simulink model "LGS_allFaultsDeselected"  (R2019b)
settings: Solver=FixedStepDiscrete  StartTime=0.0  StopTime=45.0  FixedStep=0.1  RelTol=1e-3
model workspace (MAT data in the model file):
  fipData{1} = [0; 0]
  fipData{2} = [0; 0]
  fipData{3} = [0; 0]
  fipData{4} = [0; 0]
  fipData{5} = [0; 0]
  fipData{6} = [0; 0]
  fipData{7} = [0; 0]
  fipData{8} = [0; 0]
  fipData{9} = [0; 0]
  fipData{10} = [0; 0]
  fipData{11} = [0; 0]
  fipData{12} = [0; 0]
  fipData{13} = [0; 0]
  fipData{14} = [0; 0]
  fipData{15} = [0; 0]
  fipData{16} = [0; 0]
  fipData{17} = [0; 0]
  fipData{18} = [0; 0]
  fipData{19} = [0; 0]
  fipData{20} = [0; 0]
  fipData{21} = [0; 0]
  fipData{22} = [0; 0]
  fipData{23} = [0; 0]
  fipData{24} = [0; 0]
  fipData{25} = [0; 0]
  fipData{26} = [0; 0]
  fipData{27} = [0; 0]
  fipData{28} = [0; 0]
  fipData{29} = [0; 0]
  fipData{30} = [0; 0]
  fipData{31} = [0; 0]
  fipData{32} = [0; 0]
  fipData{33} = [0; 0]
  fipData{34} = [0; 0]
  fipData{35} = [0; 0]
  fipData{36} = [0; 0]
  fipData{37} = [0; 0]
  fipData{38} = [0; 0]
  fipData{39} = [0; 0]
  fipData{40} = [0; 0]
  fipData{41} = [0; 0]
  fipData{42} = [0; 0]
  fipData{43} = [0; 0]
  fipData{44} = [0; 0]
  fipData{45} = [0; 0]
  fipData{46} = [0; 0]
  fipData{47} = [0; 0]
  fipData{48} = [0; 0]
  fipData{49} = [0; 0]
  fipData{50} = [0; 0]
  fipData{51} = [0; 0]
  fipData{52} = [0; 0]
  fipData{53} = [0; 0]
  fipData{54} = [0; 0]
  fipData{55} = [0; 0]
  fipData{56} = [0; 0]
  fipData{57} = [0; 0]
  fipData{58} = [0; 0]
  fipData{59} = [0; 0]
  fipData{60} = [0; 0]
  fipData{61} = [0; 0]
  fipData{62} = [0; 0]
  fipData{63} = [0; 0]
  fipData{64} = [0; 0]
  fipData{65} = [0; 0]
  fipData{66} = [0; 0]
  fipData{67} = [0; 0]
  fipData{68} = [0; 0]
  fipData{69} = [0; 0]
  fipData{70} = [0; 0]
  fipData{71} = [0; 0]
  fipData{72} = [0; 0]
  fipData{73} = [0; 0]
  fipData{74} = [0; 0]
  fipData{75} = [0; 0]
  fipData{76} = [0; 0]
  fipData{77} = [0; 0]
  fipData{78} = [0; 0]
  fipData{79} = [0; 0]
  fipData{80} = [0; 0]
  fipData{81} = [0; 0]
  fipData{82} = [0; 0]
  fipData{83} = [0; 0]
  fipData{84} = [0; 0]
  fipData{85} = [0; 0]
  fipData{86} = [0; 0]
  fipData{87} = [0; 0]
  fipData{88} = [0; 0]
  fipData{89} = [0; 0]
  fipData{90} = [0; 0]
  fipData{91} = [0; 0]
  fipData{92} = [0; 0]
  fipData{93} = [0; 0]
  fipData{94} = [0; 0]
  fipData{95} = [0; 0]
  fipData{96} = [0; 0]
  fipData{97} = [0; 0]
  fipData{98} = [0; 0]
  fipData{99} = [0; 0]
  fipData{100} = [0; 0]
  fipData{101} = [0; 0]
  fipData{102} = [0; 0]
  fipData{103} = [0; 0]
  fipData{104} = [0; 0]
  fipData{105} = [0; 0]
  fipData{106} = [0; 0]
  fipData{107} = [0; 0]
  fipData{108} = [0; 0]
  fipData{109} = [0; 0]
  fipData{110} = [0; 0]
  fipData{111} = [0; 0]
  fipData{112} = [0; 0]
  fipData{113} = [0; 0]
  fipData{114} = [0; 0]
  fipData{115} = [0; 0]
  fipData{116} = [0; 0]
  fipData{117} = [0; 0]
  fipData{118} = [0; 0]
  fipData{119} = [0; 0]
  fipData{120} = [0; 0]
  fipData{121} = [0; 0]
  fipData{122} = [0; 0]
  fipData{123} = [0; 0]
  fipData{124} = [0; 0]
  fipData{125} = [0; 0]
  fipData{126} = [0; 0]
  fipData{127} = [0; 0]
  fipData{128} = [0; 0]
  fipData{129} = [0; 0]
  fipData{130} = [0; 0]
  fipData{131} = [0; 0]
  fipData{132} = [0; 0]
  fipData{133} = [0; 0]
  fipData{134} = [0; 0]
  fipData{135} = [0; 0]
  fipData{136} = [0; 0]
  fipData{137} = [0; 0]
  fipData{138} = [0; 0]
  fipData{139} = [0; 0]
  fipData{140} = [0; 0]
  fipData{141} = [0; 0]
  fipData{142} = [0; 0]
  fipData{143} = [0; 0]
  fipData{144} = [0; 0]
  fipData{145} = [0; 0]
  fipData{146} = [0; 0]
  fipData{147} = [0; 0]
  fipData{148} = [0; 0]
  fipData{149} = [0; 0]
  fipData{150} = [0; 0]
  fipData{151} = [0; 0]
  fipData{152} = [0; 0]
  fipData{153} = [0; 0]
  fipData{154} = [0; 0]
  fipData{155} = [0; 0]
  fipData{156} = [0; 0]
  fipData{157} = [0; 0]
  fipData{158} = [0; 0]
  fipData{159} = [0; 0]
  fipData{160} = [0; 0]
  fipData{161} = [0; 0]
  fipData{162} = [0; 0]
  fipData{163} = [0; 0]
  fipData{164} = [0; 0]
  fipData{165} = [0; 0]
  fipData{166} = [0; 0]
  fipData{167} = [0; 0]
  fipData{168} = [0; 0]
  fipData{169} = [0; 0]
  fipData{170} = [0; 0]
  fipData{171} = [0; 0]
  fipData{172} = [0; 0]
  fipData{173} = [0; 0]
  fipData{174} = [0; 0]
  fipData{175} = [0; 0]
  fipData{176} = [0; 0]
  fipData{177} = [0; 0]
  fipData{178} = [0; 0]
  fipData{179} = [0; 0]
  fipData{180} = [0; 0]
  fipData{181} = [0; 0]
  fipData{182} = [0; 0]
  fipData{183} = [0; 0]
  fipData{184} = [0; 0]
  fipData{185} = [0; 0]
  fipData{186} = [0; 0]
  fipData{187} = [0; 0]
  fipData{188} = [0; 0]
  fipData{189} = [0; 0]
  fipData{190} = [0; 0]
  fipData{191} = [0; 0]
  fipData{192} = [0; 0]
  fipData{193} = [0; 0]
  fipData{194} = [0; 0]
  fipData{195} = [0; 0]
  fipData{196} = [0; 0]
  fipData{197} = [0; 0]
  fipData{198} = [0; 0]
  fipData{199} = [0; 0]
  fipData{200} = [0; 0]
  fipData{201} = [0; 0]
  fipData{202} = [0; 0]
  fipData{203} = [0; 0]
  fipData{204} = [0; 0]
  fipData{205} = [0; 0]
  fipData{206} = [0; 0]
  fipData{207} = [0; 0]
  fipData{208} = [0; 0]
  fipData{209} = [0; 0]
  fipData{210} = [0; 0]
  fipData{211} = [0; 0]
  fipData{212} = [0; 0]
  fipData{213} = [0; 0]
  fipData{214} = [0; 0]
  fipData{215} = [0; 0]
  fipData{216} = [0; 0]
  fipData{217} = [0; 0]
  fipData{218} = [0; 0]
  fipData{219} = [0; 0]
  fipData{220} = [0; 0]
  fipData{221} = [0; 0]
  fipData{222} = [0; 0]
  fipData{223} = [0; 0]
  fipData{224} = [0; 0]
  fipData{225} = [0; 0]
  fipData{226} = [0; 0]
  fipData{227} = [0; 0]
  fipData{228} = [0; 0]
  fipData{229} = [0; 0]
  fipData{230} = [0; 0]
  fipData{231} = [0; 0]
  fipData{232} = [0; 0]
  fipData{233} = [0; 0]
  fipData{234} = [0; 0]
  fipData{235} = [0; 0]
  fipData{236} = [0; 0]
  fipData{237} = [0; 0]
  fipData{238} = [0; 0]
  fipData{239} = [0; 0]
  fipData{240} = [0; 0]
  fipData{241} = [0; 0]
  fipData{242} = [0; 0]
  fipData{243} = [0; 0]
  fipData{244} = [0; 0]
  fipData{245} = [0; 0]
  fipData{246} = [0; 0]
  fipData{247} = [0; 0]
  fipData{248} = [0; 0]
  fipData{249} = [0; 0]
  fipData{250} = [0; 0]
  fipData{251} = [0; 0]
  fipData{252} = [0; 0]
  fipData{253} = [0; 0]
  fipData{254} = [0; 0]
  fipName : object (value not decoded)
  stepSize = 0.1
libraries: LibFaultInjectionControls x190, commrandsrc3 x70, simulink x3, LibFailureCondition x1
(part 1 of 41)
settings Model: LastInjection=18-Mar-2021 09:43:28  Creator=wiebk  LastModifiedBy=Hannes Stuetzer
settings DataIOCC: ReturnWorkspaceOutputs=off
settings DebuggingCC: ArithmeticOperatorsInVariantConditions=warning
settings SFSimCC: SimUseLocalCustomCode=off  CustomCodeUndefinedFunction=UseInterfaceOnly
settings RTWCC: RTWUseLocalCustomCode=off
settings CodeAppCC: StateflowObjectComments=on
settings ConfigComp: DVMode=PropertyProving  DVMaxProcessTime=30000  DVAutomaticStubbing=off  DVParameters=on  DVParametersUseConfig=on  DVModelCoverageObjectives=None  DVMaxTestCaseSteps=1  DVTestSuiteOptimization=CombinedObjectives (Nonlinear Extended)

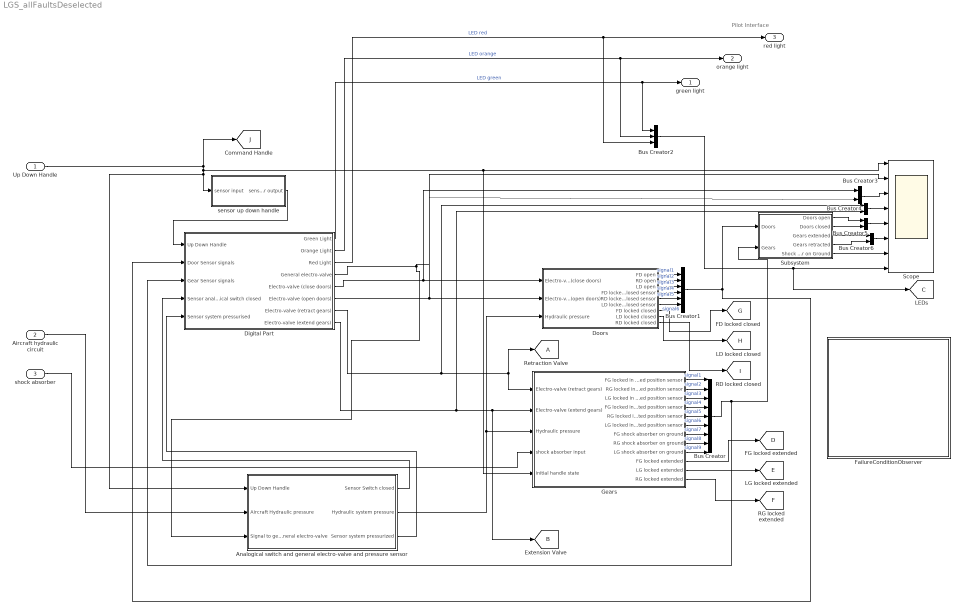
== system LGS_allFaultsDeselected ==
  note: Pilot Interface
  Up Down Handle : Inport  OutDataTypeStr=boolean  SampleTime=0.1
  Aircraft hydraulic circuit : Inport  Port=2  OutDataTypeStr=boolean  SampleTime=0.1
  shock absorber : Inport  Port=3  OutDataTypeStr=boolean  SampleTime=0.1
  Analogical switch and general electro-valve and pressure sensor : Subsystem
  Bus Creator : BusCreator  Inputs=9
  Bus Creator1 : BusCreator  Inputs=6
  Bus Creator2 : BusCreator  Inputs=3
  Bus Creator{3..6} (4 alike) : BusCreator  Inputs=2
  Digital Part : Subsystem
  Doors : Subsystem
  FailureConditionObserver : Subsystem  AncestorBlock=LibFailureCondition/FailureConditionObserver  InitFcn=|  mask(FailureConditionObserver){Parameter2=0}
      | pathName = gcb;
      | f = Simulink.FindOptions('SearchDepth',4);
      | blocks = Simulink.findBlocks(gcb,f);
      | for i=1:length(blocks)
      |     if get_param(blocks(i), 'StaticLinkStatus') == "resolved"
      |         disp( get_param(blocks(i), 'StaticLinkStatus'));
      |         set_param(blocks(i),'LinkStatus','inactive');
      |      end
      | end
      mask help: FailureConditionObserver
      mask init:
      | fch = FailureConditionHelper;
      | disp(fch.checkForFailureConditionObserver(gcb))
      | if 1 < fch.checkForFailureConditionObserver(gcb)
      |     errordlg("This is not the first FailureConditionObserver within this model. Please ensure that only one FailureConditionObserver resides within a midel.")
      | end
      | 
      | pathName = gcb;
      | f = Simulink.FindOptions('SearchDepth',4);
      | set_param(gcb,'LinkStatus','inactive');
      | blocks = Simulink.findBlocks(gcb,f);
      | for i=1:length(blocks)
      |     if get_param(blocks(i), 'StaticLinkStatus') == "resolved"
      |         if not(contains(get_param(blocks(i), 'Name'), 'DiveObserver'))
      |             set_param(blocks(i),'LinkStatus','inactive');
      |         end
      | 
      |     end
      | end
      mask Help: FailureConditionObserver
      mask Callback Parameter2:
      | fch = FailureConditionHelper;
      | disp(fch.checkForFailureConditionObserver(gcb))
      | if 1 < fch.checkForFailureConditionObserver(gcb)
      |     errordlg("This is not the first FailureConditionObserver within this model. Please ensure that only one FailureConditionObserver resides within a midel.")
      | end
      mask Display: image('failurecondition.png'); % Use "Edit Image" on toolstrip to change.
  Gears : Subsystem
  Scope : Scope  NumInputPorts=8
  Subsystem : Subsystem
  sensor up down handle : Subsystem
  green light : Outport  OutDataTypeStr=boolean  SampleTime=0.1
  orange light : Outport  Port=2  OutDataTypeStr=boolean  SampleTime=0.1
  red light : Outport  Port=3  OutDataTypeStr=boolean  SampleTime=0.1
  tag scope: A=global, B=global, C=global, D=global, E=global, F=global, G=global, H=global, I=global, J=global
  wires:
  sensor up down handle/1(sensor output) -> Digital Part/1(Up Down Handle)
  Analogical switch and general electro-valve and pressure sensor/2(Hydraulic system pressure) -> Gears/3(Hydraulic pressure), Doors/3(Hydraulic pressure)
  Gears/1(FG locked in extended position sensor) -> Bus Creator/1  "signal1"
  Gears/2(RG locked in extended position sensor) -> Bus Creator/2  "signal2"
  Gears/3(LG locked in extended position sensor) -> Bus Creator/3  "signal3"
  Gears/4(FG locked in retracted position sensor) -> Bus Creator/4  "signal4"
  Gears/5(RG locked in retracted position sensor) -> Bus Creator/5  "signal5"
  Gears/6(LG locked in retracted position sensor) -> Bus Creator/6  "signal6"
  Gears/7(FG shock absorber on ground) -> Bus Creator/7  "signal7"
  Gears/8(RG shock absorber on ground) -> Bus Creator/8  "signal8"
  Gears/9(LG shock absorber on ground) -> Bus Creator/9  "signal9"
  Doors/1(FD open) -> Bus Creator1/1  "signal1"
  Doors/2(RD open) -> Bus Creator1/2  "signal2"
  Doors/3(LD open) -> Bus Creator1/3  "signal3"
  Doors/4(FD locked closed sensor) -> Bus Creator1/4  "signal4"
  Doors/5(RD locked closed sensor) -> Bus Creator1/5  "signal5"
  Doors/6(LD locked closed sensor) -> Bus Creator1/6  "signal6"
  Bus Creator1/1 -> Digital Part/2(Door Sensor signals), Subsystem/1(Doors)
  Analogical switch and general electro-valve and pressure sensor/1(Sensor Switch closed) -> Digital Part/4(Sensor analogical switch closed)
  Analogical switch and general electro-valve and pressure sensor/3(Sensor system pressurized) -> Digital Part/5(Sensor system pressurised)
  Bus Creator/1 -> Digital Part/3(Gear Sensor signals), Subsystem/2(Gears)
  Subsystem/1(Doors open) -> Bus Creator5/1
  Subsystem/2(Doors closed) -> Bus Creator5/2
  Bus Creator3/1 -> Scope/3
  Bus Creator4/1 -> Scope/4
  Bus Creator5/1 -> Scope/5
  Bus Creator6/1 -> Scope/6
  Subsystem/3(Gears extended) -> Bus Creator6/1
  Subsystem/4(Gears retracted) -> Bus Creator6/2
  Subsystem/5(Shock Obserber on Ground) -> Scope/7
  Bus Creator2/1 -> [C], Scope/8
  Digital Part/4(General electro-valve) -> Analogical switch and general electro-valve and pressure sensor/3(Signal to general electro-valve), Scope/2
  Digital Part/1(Green Light) -> Bus Creator2/1, green light/1  "LED green"
  Digital Part/2(Orange Light) -> Bus Creator2/2, orange light/1  "LED orange"
  Digital Part/3(Red Light) -> Bus Creator2/3, red light/1  "LED red"
  Aircraft hydraulic circuit/1 -> Analogical switch and general electro-valve and pressure sensor/2(Aircraft Hydraulic pressure)
  Digital Part/8(Electro-valve (extend gears)) -> Bus Creator4/2, [B], Gears/2(Electro-valve (extend gears))
  Digital Part/7(Electro-valve (retract gears)) -> Bus Creator4/1, [A], Gears/1(Electro-valve (retract gears))
  Digital Part/6(Electro-valve (open doors)) -> Bus Creator3/2, Doors/2(Electro-valve (open doors))
  Digital Part/5(Electro-valve (close doors)) -> Bus Creator3/1, Doors/1(Electro-valve (close doors))
  Up Down Handle/1 -> [J], Scope/1, Gears/5(initial handle state), Analogical switch and general electro-valve and pressure sensor/1(Up Down Handle), sensor up down handle/1(sensor input)
  shock absorber/1 -> Gears/4(shock absorber input)
  Gears/10(FG locked extended) -> [D]
  Gears/11(LG locked extended) -> [E]
  Gears/12(RG locked extended) -> [F]
  Doors/7(FD locked closed) -> [G]
  Doors/8(LD locked closed) -> [H]
  Doors/9(RD locked closed) -> [I]

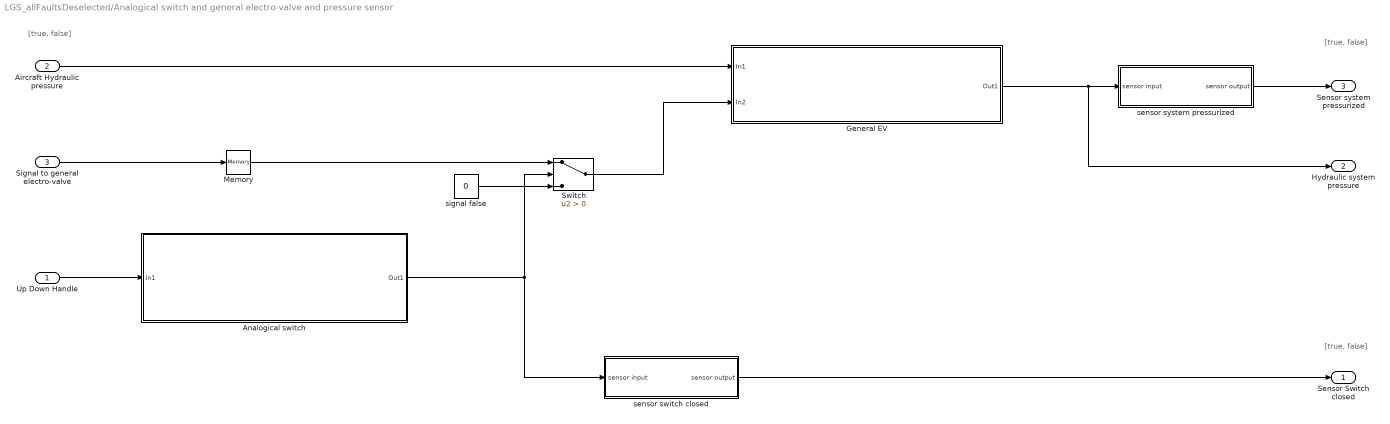
== system LGS_allFaultsDeselected/Analogical switch and general electro-valve and pressure sensor ==
  note: [true, false]
  note: [true, false]
  note: [true, false]
  Up Down Handle : Inport  OutDataTypeStr=boolean
  Aircraft Hydraulic pressure : Inport  Port=2  OutDataTypeStr=boolean
  Signal to general electro-valve : Inport  Port=3  OutDataTypeStr=boolean
  Analogical switch : Subsystem
  General EV : Subsystem
  Memory : Memory  InheritSampleTime=on
  Switch : Switch  Criteria=u2 > Threshold
  sensor switch closed : Subsystem
  sensor system pressurized : Subsystem
  signal false : Constant  Value=0  OutDataTypeStr=boolean
  Sensor Switch closed : Outport
  Hydraulic system pressure : Outport  Port=2  OutDataTypeStr=boolean
  Sensor system pressurized : Outport  Port=3
  wires:
  Up Down Handle/1 -> Analogical switch/1(In1)
  Aircraft Hydraulic pressure/1 -> General EV/1(In1)
  signal false/1 -> Switch/3
  Signal to general electro-valve/1 -> Memory/1
  Switch/1 -> General EV/2(In2)
  Analogical switch/1(Out1) -> Switch/2, sensor switch closed/1(sensor input)
  sensor switch closed/1(sensor output) -> Sensor Switch closed/1
  General EV/1(Out1) -> Hydraulic system pressure/1, sensor system pressurized/1(sensor input)
  sensor system pressurized/1(sensor output) -> Sensor system pressurized/1
  Memory/1 -> Switch/1

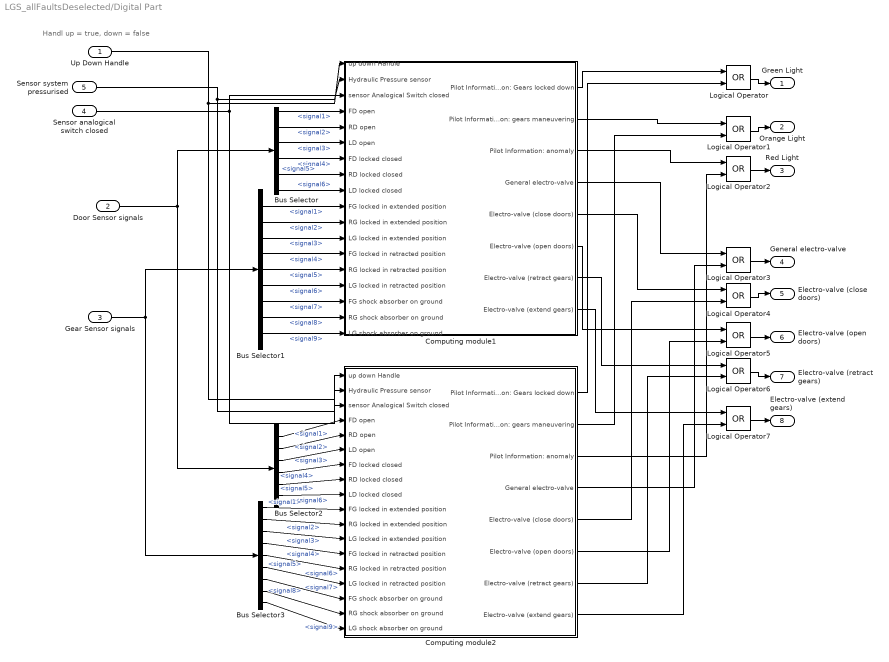
== system LGS_allFaultsDeselected/Digital Part ==
  note: Handl up = true, down = false
  Up Down Handle : Inport
  Door Sensor signals : Inport  Port=2
  Gear Sensor signals : Inport  Port=3
  Sensor analogical switch closed : Inport  Port=4
  Sensor system pressurised : Inport  Port=5
  Bus Selector : BusSelector  OutputSignals=signal1,signal2,signal3,signal4,signal5,signal6
  Bus Selector1 : BusSelector  OutputSignals=signal1,signal2,signal3,signal4,signal5,signal6,signal7,signal8,signal9
  Bus Selector2 : BusSelector  OutputSignals=signal1,signal2,signal3,signal4,signal5,signal6
  Bus Selector3 : BusSelector  OutputSignals=signal1,signal2,signal3,signal4,signal5,signal6,signal7,signal8,signal9
  Computing module1 : Subsystem
  Computing module2 : Subsystem
  Logical Operator{,1..7} (8 alike) : Logic  Operator=OR  AllPortsSameDT=off  OutDataTypeStr=boolean
  Green Light : Outport  OutDataTypeStr=boolean
  Orange Light : Outport  Port=2  OutDataTypeStr=boolean
  Red Light : Outport  Port=3  OutDataTypeStr=boolean
  General electro-valve : Outport  Port=4  OutDataTypeStr=boolean
  Electro-valve (close doors) : Outport  Port=5  OutDataTypeStr=boolean
  Electro-valve (open doors) : Outport  Port=6  OutDataTypeStr=boolean
  Electro-valve (retract gears) : Outport  Port=7  OutDataTypeStr=boolean
  Electro-valve (extend gears) : Outport  Port=8  OutDataTypeStr=boolean
  wires:
  Door Sensor signals/1 -> Bus Selector2/1, Bus Selector/1
  Gear Sensor signals/1 -> Bus Selector3/1, Bus Selector1/1
  Up Down Handle/1 -> Computing module2/1(up down Handle), Computing module1/1(up down Handle)
  Sensor system pressurised/1 -> Computing module2/2(Hydraulic Pressure sensor), Computing module1/2(Hydraulic Pressure sensor)
  Sensor analogical switch closed/1 -> Computing module2/3(" sensor Analogical Switch closed"), Computing module1/3(" sensor Analogical Switch closed")
  Computing module1/1(Pilot Information: Gears locked down) -> Logical Operator/1
  Bus Selector/1 -> Computing module1/4(FD open)  "<signal1>"
  Bus Selector/6 -> Computing module1/9(LD locked closed)  "<signal6>"
  Bus Selector1/1 -> Computing module1/10(FG locked in extended position)  "<signal1>"
  Bus Selector1/2 -> Computing module1/11(RG locked in extended position)  "<signal2>"
  Bus Selector1/3 -> Computing module1/12(LG locked in extended position)  "<signal3>"
  Bus Selector1/4 -> Computing module1/13(FG locked in retracted position)  "<signal4>"
  Bus Selector1/5 -> Computing module1/14(RG locked in retracted position)  "<signal5>"
  Bus Selector1/6 -> Computing module1/15(LG locked in retracted position)  "<signal6>"
  Bus Selector1/7 -> Computing module1/16(FG shock absorber on ground)  "<signal7>"
  Bus Selector1/8 -> Computing module1/17(RG shock absorber on ground)  "<signal8>"
  Bus Selector1/9 -> Computing module1/18(LG shock absorber on ground)  "<signal9>"
  Computing module1/3(Pilot Information: anomaly) -> Logical Operator2/1
  Computing module1/4(General electro-valve) -> Logical Operator3/1
  Computing module1/5(Electro-valve (close doors)) -> Logical Operator4/1
  Computing module1/6(Electro-valve (open doors)) -> Logical Operator5/1
  Computing module1/7(Electro-valve (retract gears)) -> Logical Operator6/1
  Computing module1/8(Electro-valve (extend gears)) -> Logical Operator7/1
  Logical Operator/1 -> Green Light/1
  Computing module1/2(Pilot Information: gears maneuvering) -> Logical Operator1/1
  Logical Operator1/1 -> Orange Light/1
  Logical Operator2/1 -> Red Light/1
  Logical Operator3/1 -> General electro-valve/1
  Logical Operator4/1 -> Electro-valve (close doors)/1
  Logical Operator5/1 -> Electro-valve (open doors)/1
  Logical Operator6/1 -> Electro-valve (retract gears)/1
  Logical Operator7/1 -> Electro-valve (extend gears)/1
  Computing module2/1(Pilot Information: Gears locked down) -> Logical Operator/2
  Computing module2/2(Pilot Information: gears maneuvering) -> Logical Operator1/2
  Computing module2/3(Pilot Information: anomaly) -> Logical Operator2/2
  Computing module2/4(General electro-valve) -> Logical Operator3/2
  Computing module2/5(Electro-valve (close doors)) -> Logical Operator4/2
  Computing module2/6(Electro-valve (open doors)) -> Logical Operator5/2
  Computing module2/7(Electro-valve (retract gears)) -> Logical Operator6/2
  Computing module2/8(Electro-valve (extend gears)) -> Logical Operator7/2
  Bus Selector2/1 -> Computing module2/4(FD open)  "<signal1>"
  Bus Selector2/2 -> Computing module2/5(RD open)  "<signal2>"
  Bus Selector2/3 -> Computing module2/6(LD open)  "<signal3>"
  Bus Selector2/4 -> Computing module2/7(FD locked closed)  "<signal4>"
  Bus Selector2/5 -> Computing module2/8(RD locked closed)  "<signal5>"
  Bus Selector2/6 -> Computing module2/9(LD locked closed)  "<signal6>"
  Bus Selector3/1 -> Computing module2/10(FG locked in extended position)  "<signal1>"
  Bus Selector3/2 -> Computing module2/11(RG locked in extended position)  "<signal2>"
  Bus Selector3/3 -> Computing module2/12(LG locked in extended position)  "<signal3>"
  Bus Selector3/4 -> Computing module2/13(FG locked in retracted position)  "<signal4>"
  Bus Selector3/5 -> Computing module2/14(RG locked in retracted position)  "<signal5>"
  Bus Selector3/6 -> Computing module2/15(LG locked in retracted position)  "<signal6>"
  Bus Selector3/7 -> Computing module2/16(FG shock absorber on ground)  "<signal7>"
  Bus Selector3/8 -> Computing module2/17(RG shock absorber on ground)  "<signal8>"
  Bus Selector3/9 -> Computing module2/18(LG shock absorber on ground)  "<signal9>"
  Bus Selector/2 -> Computing module1/5(RD open)  "<signal2>"
  Bus Selector/3 -> Computing module1/6(LD open)  "<signal3>"
  Bus Selector/4 -> Computing module1/7(FD locked closed)  "<signal4>"
  Bus Selector/5 -> Computing module1/8(RD locked closed)  "<signal5>"

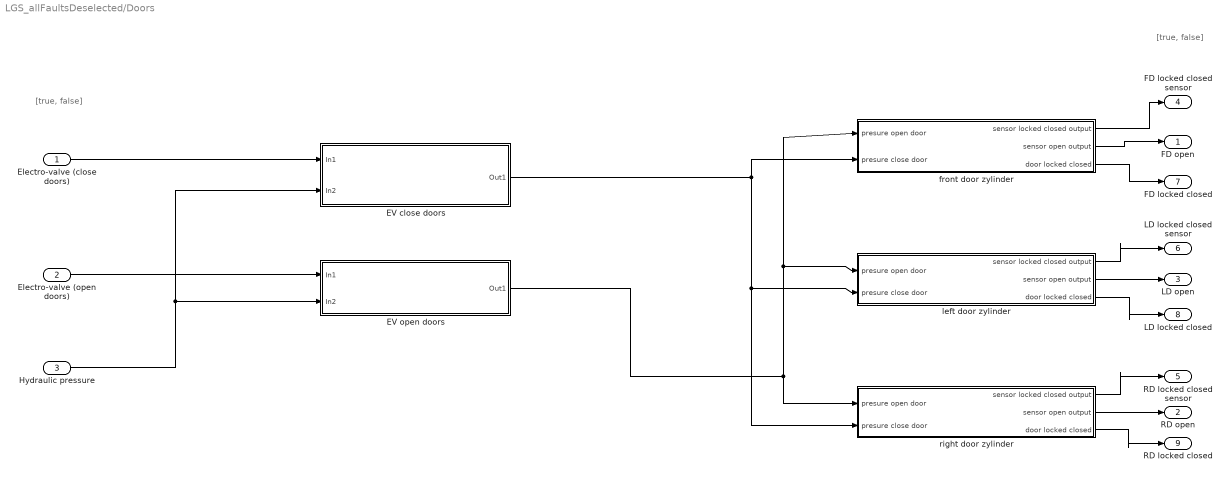
== system LGS_allFaultsDeselected/Doors ==
  note: [true, false]
  note: [true, false]
  Electro-valve (close doors) : Inport  OutDataTypeStr=boolean
  Electro-valve (open doors) : Inport  Port=2  OutDataTypeStr=boolean
  Hydraulic pressure : Inport  Port=3  OutDataTypeStr=boolean
  EV close doors : Subsystem
  EV open doors : Subsystem
  front door zylinder : Subsystem
  left door zylinder : Subsystem
  right door zylinder : Subsystem
  FD open : Outport
  RD open : Outport  Port=2
  LD open : Outport  Port=3
  FD locked closed sensor : Outport  Port=4
  RD locked closed sensor : Outport  Port=5
  LD locked closed sensor : Outport  Port=6
  FD locked closed : Outport  Port=7
  LD locked closed : Outport  Port=8
  RD locked closed : Outport  Port=9
  wires:
  Hydraulic pressure/1 -> EV close doors/2(In2), EV open doors/2(In2)
  front door zylinder/1(sensor locked closed output) -> FD locked closed sensor/1
  front door zylinder/2(sensor open output) -> FD open/1
  left door zylinder/2(sensor open output) -> LD open/1
  left door zylinder/1(sensor locked closed output) -> LD locked closed sensor/1
  right door zylinder/1(sensor locked closed output) -> RD locked closed sensor/1
  right door zylinder/2(sensor open output) -> RD open/1
  EV close doors/1(Out1) -> right door zylinder/2(presure close door), left door zylinder/2(presure close door), front door zylinder/2(presure close door)
  EV open doors/1(Out1) -> right door zylinder/1(presure open door), left door zylinder/1(presure open door), front door zylinder/1(presure open door)
  Electro-valve (close doors)/1 -> EV close doors/1(In1)
  Electro-valve (open doors)/1 -> EV open doors/1(In1)
  front door zylinder/3(door locked closed) -> FD locked closed/1
  left door zylinder/3(door locked closed) -> LD locked closed/1
  right door zylinder/3(door locked closed) -> RD locked closed/1

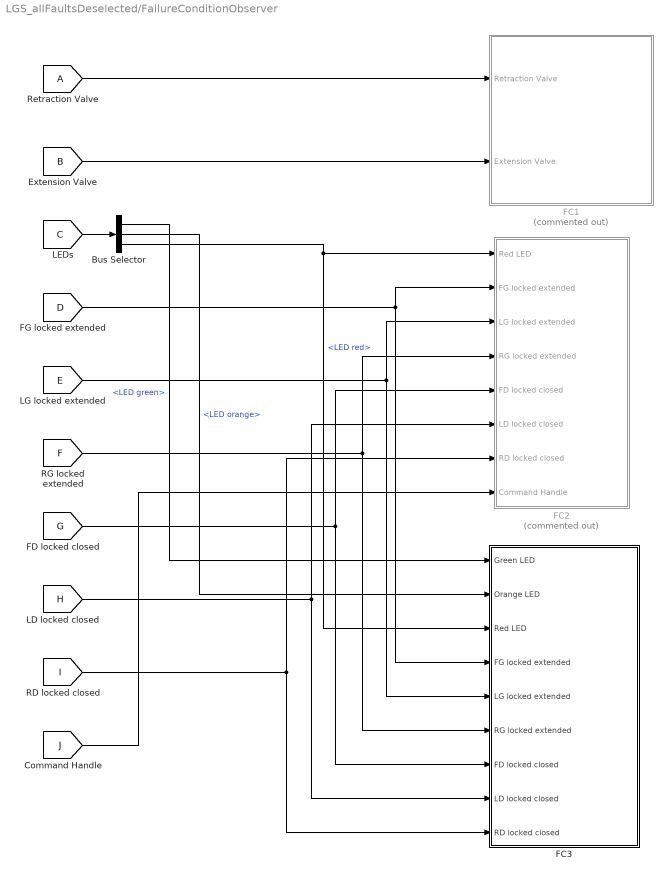
== system LGS_allFaultsDeselected/FailureConditionObserver ==
  Bus Selector : BusSelector  OutputSignals=LED green,LED orange,LED red
  FC1 : Subsystem  Commented=on  AncestorBlock=LibFailureCondition/FailureCondition  mask(FailureCondition){ID=FC1, Details=Simultaneous outgoing and retraction, Criticality=catastrophic, SafetyTarget=1E-9, DesignTarget=0, Parameter5=}
      mask prompts: SafetyTarget "Safety Target"; DesignTarget "Design Target"
      mask help: FailureCondition
      mask Help: FailureCondition
      mask Callback ID:
      | id = get_param(gcb, 'ID')
      | set_param(gcb, 'name', id)
      mask TypeOptions Criticality: no safety effect | minor | major | hazardous | catastrophic
      mask Callback Criticality:
      | c = get_param(gcb, 'Criticality');
      | 
      | disp(c)
      | switch(c)
      |    case 'catastrophic'
      |       set_param(gcb, 'SafetyTarget', '1E-9');
      |    case 'hazardous'
      |       set_param(gcb, 'SafetyTarget', '1E-7');
      |    case 'major'
      |       set_param(gcb, 'SafetyTarget', '1E-5');
      |    case 'minor'
      |       set_param(gcb, 'SafetyTarget', '1E-3');
      |    case 'no safety effect'
      |       set_param(gcb, 'SafetyTarget', '0');
      |    otherwise
      |       set_param(gcb, 'SafetyTarget', '-1');
      | end
      mask DialogControl Details Tooltip: Insert the description of the Failure Condition here.
      mask DialogControl Criticality Tooltip: Choose the criticality of the failure condition. The risk value is set automatically according to the defined value.
      mask DialogControl SafetyTarget Tooltip: This value is derived from the given criticality. It specifies the safety target for the quantitative analysis.
      mask DialogControl DesignTarget Tooltip: Specify a design target for the quantitative analysis.
      mask DialogControl Container4 Prompt: Notes
  FC2 : Subsystem  Commented=on  AncestorBlock=LibFailureCondition/FailureCondition  mask(FailureCondition){ID=FC2, Details=15s after handle has been pushed to extension position and not moved again, gears are not locked extended or doors closed, Criticality=hazardous, SafetyTarget=1E-7, DesignTarget=0, Parameter5=}
      mask prompts: SafetyTarget "Safety Target"; DesignTarget "Design Target"
      mask help: FailureCondition
      mask Help: FailureCondition
      mask Callback ID:
      | id = get_param(gcb, 'ID')
      | set_param(gcb, 'name', id)
      mask TypeOptions Criticality: no safety effect | minor | major | hazardous | catastrophic
      mask Callback Criticality:
      | c = get_param(gcb, 'Criticality');
      | 
      | disp(c)
      | switch(c)
      |    case 'catastrophic'
      |       set_param(gcb, 'SafetyTarget', '1E-9');
      |    case 'hazardous'
      |       set_param(gcb, 'SafetyTarget', '1E-7');
      |    case 'major'
      |       set_param(gcb, 'SafetyTarget', '1E-5');
      |    case 'minor'
      |       set_param(gcb, 'SafetyTarget', '1E-3');
      |    case 'no safety effect'
      |       set_param(gcb, 'SafetyTarget', '0');
      |    otherwise
      |       set_param(gcb, 'SafetyTarget', '-1');
      | end
      mask DialogControl Details Tooltip: Insert the description of the Failure Condition here.
      mask DialogControl Criticality Tooltip: Choose the criticality of the failure condition. The risk value is set automatically according to the defined value.
      mask DialogControl SafetyTarget Tooltip: This value is derived from the given criticality. It specifies the safety target for the quantitative analysis.
      mask DialogControl DesignTarget Tooltip: Specify a design target for the quantitative analysis.
      mask DialogControl Container4 Prompt: Notes
  FC3 : Subsystem  AncestorBlock=LibFailureCondition/FailureCondition  mask(FailureCondition){ID=FC3, Details=Hello: Gear is not locked down althoug implied by monitoring LEDs, Criticality=major, SafetyTarget=1E-5, DesignTarget=6e-9, Parameter5=Tim}
      mask prompts: SafetyTarget "Safety Target"; DesignTarget "Design Target"
      mask help: FailureCondition
      mask Help: FailureCondition
      mask Callback ID:
      | id = get_param(gcb, 'ID')
      | set_param(gcb, 'name', id)
      mask TypeOptions Criticality: no safety effect | minor | major | hazardous | catastrophic
      mask Callback Criticality:
      | c = get_param(gcb, 'Criticality');
      | 
      | disp(c)
      | switch(c)
      |    case 'catastrophic'
      |       set_param(gcb, 'SafetyTarget', '1E-9');
      |    case 'hazardous'
      |       set_param(gcb, 'SafetyTarget', '1E-7');
      |    case 'major'
      |       set_param(gcb, 'SafetyTarget', '1E-5');
      |    case 'minor'
      |       set_param(gcb, 'SafetyTarget', '1E-3');
      |    case 'no safety effect'
      |       set_param(gcb, 'SafetyTarget', '0');
      |    otherwise
      |       set_param(gcb, 'SafetyTarget', '-1');
      | end
      mask DialogControl Details Tooltip: Insert the description of the Failure Condition here.
      mask DialogControl Criticality Tooltip: Choose the criticality of the failure condition. The risk value is set automatically according to the defined value.
      mask DialogControl SafetyTarget Tooltip: This value is derived from the given criticality. It specifies the safety target for the quantitative analysis.
      mask DialogControl DesignTarget Tooltip: Specify a design target for the quantitative analysis.
      mask DialogControl Container4 Prompt: Notes
  wires:
  [C] -> Bus Selector/1
  [B] -> FC1/2(Extension Valve)
  [A] -> FC1/1(Retraction Valve)
  Bus Selector/1 -> FC3/1(Green LED)  "<LED green>"
  Bus Selector/3 -> FC3/3(Red LED), FC2/1(Red LED)  "<LED red>"
  [D] -> FC2/2(FG locked extended), FC3/4(FG locked extended)
  [E] -> FC3/5(LG locked extended), FC2/3("LG locked extended ")
  [F] -> FC3/6(RG locked extended), FC2/4(RG locked extended)
  [G] -> FC3/7(FD locked closed), FC2/5(FD locked closed)
  [H] -> FC3/8(LD locked closed), FC2/6(LD locked closed)
  [I] -> FC3/9(RD locked closed), FC2/7(RD locked closed)
  [J] -> FC2/8(Command Handle)
  Bus Selector/2 -> FC3/2(Orange LED)  "<LED orange>"

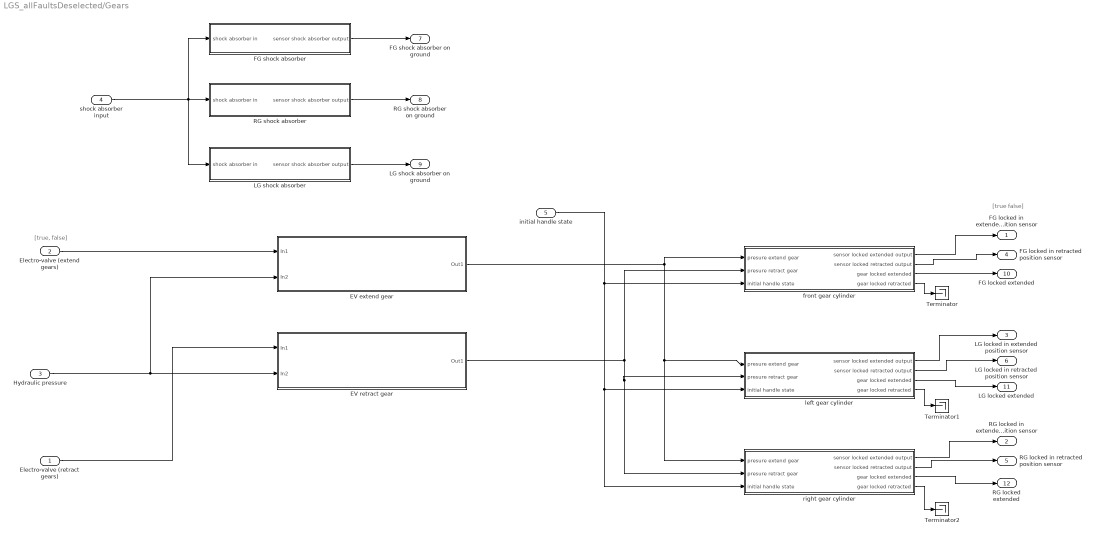
== system LGS_allFaultsDeselected/Gears ==
  note: [true, false]
  note: [true false]
  Electro-valve (retract gears) : Inport  OutDataTypeStr=boolean
  Electro-valve (extend gears) : Inport  Port=2  OutDataTypeStr=boolean
  Hydraulic pressure : Inport  Port=3  OutDataTypeStr=boolean
  shock absorber input : Inport  Port=4  OutDataTypeStr=boolean
  initial handle state : Inport  Port=5
  EV extend gear : Subsystem
  EV retract gear : Subsystem
  FG shock absorber : Subsystem
  LG shock absorber : Subsystem
  RG shock absorber : Subsystem
  Terminator : Terminator
  Terminator1 : Terminator
  Terminator2 : Terminator
  front gear cylinder : Subsystem
  left gear cylinder : Subsystem
  right gear cylinder : Subsystem
  FG locked in extended position sensor : Outport
  RG locked in extended position sensor : Outport  Port=2
  LG locked in extended position sensor : Outport  Port=3
  FG locked in retracted position sensor : Outport  Port=4
  RG locked in retracted position sensor : Outport  Port=5
  LG locked in retracted position sensor : Outport  Port=6
  FG shock absorber on ground : Outport  Port=7
  RG shock absorber on ground : Outport  Port=8
  LG shock absorber on ground : Outport  Port=9
  FG locked extended : Outport  Port=10
  LG locked extended : Outport  Port=11
  RG locked extended : Outport  Port=12
  wires:
  FG shock absorber/1(sensor shock absorber output) -> FG shock absorber on ground/1
  RG shock absorber/1(sensor shock absorber output) -> RG shock absorber on ground/1
  LG shock absorber/1(sensor shock absorber output) -> LG shock absorber on ground/1
  front gear cylinder/2(sensor locked retracted output) -> FG locked in retracted position sensor/1
  front gear cylinder/1(sensor locked extended output) -> FG locked in extended position sensor/1
  EV extend gear/1(Out1) -> front gear cylinder/1(presure extend gear), right gear cylinder/1(presure extend gear), left gear cylinder/1(presure extend gear)
  EV retract gear/1(Out1) -> right gear cylinder/2(presure retract gear), left gear cylinder/2(presure retract gear), front gear cylinder/2(presure retract gear)
  right gear cylinder/1(sensor locked extended output) -> RG locked in extended position sensor/1
  right gear cylinder/2(sensor locked retracted output) -> RG locked in retracted position sensor/1
  left gear cylinder/1(sensor locked extended output) -> LG locked in extended position sensor/1
  left gear cylinder/2(sensor locked retracted output) -> LG locked in retracted position sensor/1
  Electro-valve (extend gears)/1 -> EV extend gear/1(In1)
  Hydraulic pressure/1 -> EV extend gear/2(In2), EV retract gear/2(In2)
  Electro-valve (retract gears)/1 -> EV retract gear/1(In1)
  shock absorber input/1 -> LG shock absorber/1(shock absorber in), RG shock absorber/1(shock absorber in), FG shock absorber/1(shock absorber in)
  front gear cylinder/3(gear locked extended) -> FG locked extended/1
  left gear cylinder/3(gear locked extended) -> LG locked extended/1
  right gear cylinder/3(gear locked extended) -> RG locked extended/1
  initial handle state/1 -> left gear cylinder/3(initial handle state), right gear cylinder/3(initial handle state), front gear cylinder/3(initial handle state)
  front gear cylinder/4(gear locked retracted) -> Terminator/1
  right gear cylinder/4(gear locked retracted) -> Terminator2/1
  left gear cylinder/4(gear locked retracted) -> Terminator1/1

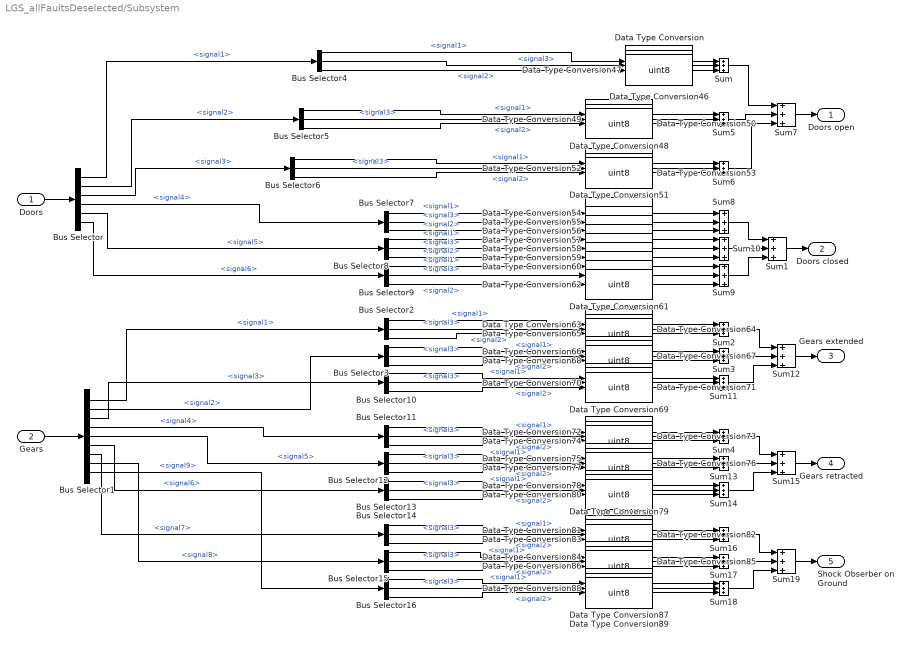
== system LGS_allFaultsDeselected/Subsystem ==
  Doors : Inport
  Gears : Inport  Port=2
  Bus Selector : BusSelector  OutputSignals=signal1,signal2,signal3,signal4,signal5,signal6
  Bus Selector1 : BusSelector  OutputSignals=signal1,signal2,signal3,signal4,signal5,signal6,signal7,signal8,signal9
  Bus Selector{2..16} (15 alike) : BusSelector  OutputSignals=signal1,signal3,signal2
  Data Type Conversion{,46..89} (45 alike) : DataTypeConversion  OutDataTypeStr=uint8
  Sum{,1..19} (20 alike) : Sum  Inputs=+++  OutDataTypeStr=int8
  Doors open : Outport  OutDataTypeStr=int8
  Doors closed : Outport  Port=2  OutDataTypeStr=int8
  Gears extended : Outport  Port=3  OutDataTypeStr=int8
  Gears retracted : Outport  Port=4  OutDataTypeStr=int8
  Shock Obserber on Ground : Outport  Port=5  OutDataTypeStr=int8
  wires:
  Bus Selector/1 -> Bus Selector4/1  "<signal1>"
  Bus Selector/2 -> Bus Selector5/1  "<signal2>"
  Bus Selector/3 -> Bus Selector6/1  "<signal3>"
  Sum/1 -> Sum7/1
  Bus Selector/4 -> Bus Selector7/1  "<signal4>"
  Bus Selector/5 -> Bus Selector8/1  "<signal5>"
  Bus Selector/6 -> Bus Selector9/1  "<signal6>"
  Sum1/1 -> Doors closed/1
  Gears/1 -> Bus Selector1/1
  Doors/1 -> Bus Selector/1
  Bus Selector4/1 -> Data Type Conversion/1  "<signal1>"
  Bus Selector4/2 -> Data Type Conversion46/1  "<signal3>"
  Bus Selector4/3 -> Data Type Conversion47/1  "<signal2>"
  Bus Selector5/1 -> Data Type Conversion48/1  "<signal1>"
  Bus Selector5/2 -> Data Type Conversion49/1  "<signal3>"
  Bus Selector5/3 -> Data Type Conversion50/1  "<signal2>"
  Bus Selector6/1 -> Data Type Conversion51/1  "<signal1>"
  Bus Selector6/2 -> Data Type Conversion52/1  "<signal3>"
  Bus Selector6/3 -> Data Type Conversion53/1  "<signal2>"
  Sum5/1 -> Sum7/2
  Sum6/1 -> Sum7/3
  Sum7/1 -> Doors open/1
  Bus Selector7/1 -> Data Type Conversion54/1  "<signal1>"
  Bus Selector7/2 -> Data Type Conversion55/1  "<signal3>"
  Bus Selector7/3 -> Data Type Conversion56/1  "<signal2>"
  Bus Selector9/2 -> Data Type Conversion61/1  "<signal3>"
  Bus Selector9/3 -> Data Type Conversion62/1  "<signal2>"
  Bus Selector9/1 -> Data Type Conversion60/1  "<signal1>"
  Bus Selector8/2 -> Data Type Conversion58/1  "<signal3>"
  Bus Selector8/3 -> Data Type Conversion59/1  "<signal2>"
  Bus Selector8/1 -> Data Type Conversion57/1  "<signal1>"
  Sum9/1 -> Sum1/3
  Sum10/1 -> Sum1/2
  Sum8/1 -> Sum1/1
  Sum2/1 -> Sum12/1
  Bus Selector2/1 -> Data Type Conversion63/1  "<signal1>"
  Bus Selector2/2 -> Data Type Conversion64/1  "<signal3>"
  Bus Selector2/3 -> Data Type Conversion65/1  "<signal2>"
  Bus Selector3/1 -> Data Type Conversion66/1  "<signal1>"
  Bus Selector3/2 -> Data Type Conversion67/1  "<signal3>"
  Bus Selector3/3 -> Data Type Conversion68/1  "<signal2>"
  Bus Selector10/1 -> Data Type Conversion69/1  "<signal1>"
  Bus Selector10/2 -> Data Type Conversion70/1  "<signal3>"
  Bus Selector10/3 -> Data Type Conversion71/1  "<signal2>"
  Sum3/1 -> Sum12/2
  Sum11/1 -> Sum12/3
  Sum12/1 -> Gears extended/1
  Bus Selector1/1 -> Bus Selector2/1  "<signal1>"
  Bus Selector1/2 -> Bus Selector3/1  "<signal2>"
  Bus Selector1/3 -> Bus Selector10/1  "<signal3>"
  Sum4/1 -> Sum15/1
  Bus Selector11/1 -> Data Type Conversion72/1  "<signal1>"
  Bus Selector11/2 -> Data Type Conversion73/1  "<signal3>"
  Bus Selector11/3 -> Data Type Conversion74/1  "<signal2>"
  Bus Selector12/1 -> Data Type Conversion75/1  "<signal1>"
  Bus Selector12/2 -> Data Type Conversion76/1  "<signal3>"
  Bus Selector12/3 -> Data Type Conversion77/1  "<signal2>"
  Bus Selector13/1 -> Data Type Conversion78/1  "<signal1>"
  Bus Selector13/2 -> Data Type Conversion79/1  "<signal3>"
  Bus Selector13/3 -> Data Type Conversion80/1  "<signal2>"
  Sum13/1 -> Sum15/2
  Sum14/1 -> Sum15/3
  Sum15/1 -> Gears retracted/1
  Sum16/1 -> Sum19/1
  Bus Selector14/1 -> Data Type Conversion81/1  "<signal1>"
  Bus Selector14/2 -> Data Type Conversion82/1  "<signal3>"
  Bus Selector14/3 -> Data Type Conversion83/1  "<signal2>"
  Bus Selector15/1 -> Data Type Conversion84/1  "<signal1>"
  Bus Selector15/2 -> Data Type Conversion85/1  "<signal3>"
  Bus Selector15/3 -> Data Type Conversion86/1  "<signal2>"
  Bus Selector16/1 -> Data Type Conversion87/1  "<signal1>"
  Bus Selector16/2 -> Data Type Conversion88/1  "<signal3>"
  Bus Selector16/3 -> Data Type Conversion89/1  "<signal2>"
  Sum17/1 -> Sum19/2
  Sum18/1 -> Sum19/3
  Sum19/1 -> Shock Obserber on Ground/1
  Bus Selector1/4 -> Bus Selector11/1  "<signal4>"
  Bus Selector1/5 -> Bus Selector12/1  "<signal5>"
  Bus Selector1/6 -> Bus Selector13/1  "<signal6>"
  Bus Selector1/7 -> Bus Selector14/1  "<signal7>"
  Bus Selector1/8 -> Bus Selector15/1  "<signal8>"
  Bus Selector1/9 -> Bus Selector16/1  "<signal9>"
  Data Type Conversion/1 -> Sum/1
  Data Type Conversion46/1 -> Sum/2
  Data Type Conversion47/1 -> Sum/3
  Data Type Conversion48/1 -> Sum5/1
  Data Type Conversion49/1 -> Sum5/2
  Data Type Conversion50/1 -> Sum5/3
  Data Type Conversion52/1 -> Sum6/2
  Data Type Conversion51/1 -> Sum6/1
  Data Type Conversion53/1 -> Sum6/3
  Data Type Conversion54/1 -> Sum8/1
  Data Type Conversion55/1 -> Sum8/2
  Data Type Conversion56/1 -> Sum8/3
  Data Type Conversion57/1 -> Sum10/1
  Data Type Conversion59/1 -> Sum10/3
  Data Type Conversion58/1 -> Sum10/2
  Data Type Conversion60/1 -> Sum9/1
  Data Type Conversion61/1 -> Sum9/2
  Data Type Conversion62/1 -> Sum9/3
  Data Type Conversion63/1 -> Sum2/1
  Data Type Conversion64/1 -> Sum2/2
  Data Type Conversion65/1 -> Sum2/3
  Data Type Conversion66/1 -> Sum3/1
  Data Type Conversion67/1 -> Sum3/2
  Data Type Conversion68/1 -> Sum3/3
  Data Type Conversion69/1 -> Sum11/1
  Data Type Conversion70/1 -> Sum11/2
  Data Type Conversion71/1 -> Sum11/3
  Data Type Conversion72/1 -> Sum4/1
  Data Type Conversion73/1 -> Sum4/2
  Data Type Conversion74/1 -> Sum4/3
  Data Type Conversion75/1 -> Sum13/1
  Data Type Conversion76/1 -> Sum13/2
  Data Type Conversion77/1 -> Sum13/3
  Data Type Conversion78/1 -> Sum14/1
  Data Type Conversion79/1 -> Sum14/2
  Data Type Conversion80/1 -> Sum14/3
  Data Type Conversion81/1 -> Sum16/1
  Data Type Conversion82/1 -> Sum16/2
  Data Type Conversion83/1 -> Sum16/3
  Data Type Conversion84/1 -> Sum17/1
  Data Type Conversion85/1 -> Sum17/2
  Data Type Conversion86/1 -> Sum17/3
  Data Type Conversion87/1 -> Sum18/1
  Data Type Conversion88/1 -> Sum18/2
  Data Type Conversion89/1 -> Sum18/3

== system LGS_allFaultsDeselected/sensor up down handle ==
  note: [true, false]
  note: [true, false]
  note: [true, false]
  sensor input : Inport
  Bus Creator3 : BusCreator  Inputs=3
  FIP1 : Subsystem
  FIP2 : Subsystem
  FIP3 : Subsystem
  sensor output : Outport
  wires:
  FIP2/1(Out1) -> Bus Creator3/2  "signal2"
  FIP1/1(Out1) -> Bus Creator3/1  "signal1"
  FIP3/1(Out1) -> Bus Creator3/3  "signal3"
  sensor input/1 -> FIP3/1(In1), FIP2/1(In1), FIP1/1(In1)
  Bus Creator3/1 -> sensor output/1

== system LGS_allFaultsDeselected/Analogical switch and general electro-valve and pressure sensor/Analogical switch ==
  In1 : Inport
  Analog Switch FIP : Subsystem  Commented=on  mask(FailureInjectionPoint){}
      mask help: FailureInjectionPoint
      mask init:
      | set_param(gcb,'LinkStatus','none');
      | 
      | treeValues = FailureInjectionPointHelper.getAllFmAndParamsAsTreeString(gcb);
      | mo = Simulink.Mask.get(gcb);
      | dc = mo.getDialogControl('GbFmInfo');
      | treeView = dc.getDialogControl('TreeViewFM');
      | treeView.TreeItems = {};
      | treeView.TreeItems = treeValues;
      settings: OpenFcn=|
      | open_system(gcb,'mask');
      | 
      | treeValues = FailureInjectionPointHelper.getAllFmAndParamsAsTreeString(gcb);
      | mo = Simulink.Mask.get(gcb);
      | dc = mo.getDialogControl('GbFmInfo');
      | treeView = dc.getDialogControl('TreeViewFM');
      | treeView.TreeItems = {};
      | treeView.TreeItems = treeValues;
      mask Help: FailureInjectionPoint
      mask DialogControl Control7 Prompt: Containing Failure Modes
      mask DialogControl BtnMoveUp Prompt: Move up
      mask DialogControl BtnMoveUp Callback:
      | %Get name of the failure mode block
      | mo = Simulink.Mask.get(gcb);
      | dc = mo.getDialogControl('GbFmInfo');
      | treeView = dc.getDialogControl('TreeViewFM');
      | try
      |     a = treeView.getSelectedItems();
      |     p = split(a, '/'); %name of failure mode block is p{1}
      | catch
      |     return;
      | end
      | 
      | %Save port handles
      | lh = get_param([gcb,'/',p{1}],'LineHandles');
      | ph = get_param([gcb,'/',p{1}],'PortHandles');
      | this_in = ph.Inport(1);
      | this_out = ph.Outport(1);
      | 
      | last_block = get_param(lh.Inport(1),'SrcBlockHandle');
      | last_block_type = get_param(last_block,'BlockType');
      | if strcmp(last_block_type,'Inport')
      |     return;
      | end
      | lb_lh = get_param(last_block,'LineHandles');
      | 
      | last_out = get_param(lh.Inport(1),'SrcPortHandle');
      | last_in = get_param(lb_lh.Inport(1),'DstPortHandle');
      | next_to_last_out = get_param(lb_lh.Inport(1),'SrcPortHandle');
      | next_in = get_param(lh.Outport(1),'DstPortHandle');
      | 
      | %Delete connecting lines
      | delete_line(lh.Inport(1));
      | delete_line(lh.Outport(1));
      | delete_line(lb_lh.Inport(1));
      | 
      | % Generate new lines
      | add_line(gcb, last_out, next_in, 'autorouting', 'smart');
      | add_line(gcb, this_out, last_in, 'autorouting', 'smart');
      | add_line(gcb, next_to_last_out, this_in, 'autorouting', 'smart');
      | 
      | %Rearrange system
      | Simulink.BlockDiagram.arrangeSystem(gcb);
      | 
      | %Refresh
      | treeValues = FailureInjectionPointHelper.getAllFmAndParamsAsTreeString(gcb);
      | mo = Simulink.Mask.get(gcb);
      | dc = mo.getDialogControl('GbFmInfo');
      | treeView = dc.getDialogControl('TreeViewFM');
      | treeView.TreeItems = {};
      | treeView.TreeItems = treeValues;
      mask DialogControl BtnMoveDown Prompt: Move down
      mask DialogControl BtnMoveDown Callback:
      | %Get name of the failure mode block
      | mo = Simulink.Mask.get(gcb);
      | dc = mo.getDialogControl('GbFmInfo');
      | treeView = dc.getDialogControl('TreeViewFM');
      | try
      |     a = treeView.getSelectedItems();
      |     p = split(a, '/'); %name of failure mode block is p{1}
      | catch
      |     return;
      | end
      | 
      | %Save port handles
      | lh = get_param([gcb,'/',p{1}],'LineHandles');
      | ph = get_param([gcb,'/',p{1}],'PortHandles');
      | this_in = ph.Inport(1);
      | this_out = ph.Outport(1);
      | 
      | next_block = get_param(lh.Outport(1),'DstBlockHandle');
      | next_block_type = get_param(next_block,'BlockType');
      | if strcmp(next_block_type,'Outport')
      |     return;
      | end
      | nb_lh = get_param(next_block,'LineHandles');
      | 
      | last_out = get_param(lh.Inport(1),'SrcPortHandle');
      | next_out = get_param(nb_lh.Outport(1),'SrcPortHandle');
      | next_but_one_in = get_param(nb_lh.Outport(1),'DstPortHandle');
      | next_in = get_param(lh.Outport(1),'DstPortHandle');
      | 
      | %Delete connecting lines
      | delete_line(lh.Inport(1));
      | delete_line(lh.Outport(1));
      | delete_line(nb_lh.Outport(1));
      | 
      | % Generate new lines
      | add_line(gcb, last_out, next_in, 'autorouting', 'smart');
      | add_line(gcb, next_out, this_in, 'autorouting', 'smart');
      | add_line(gcb, this_out, next_but_one_in, 'autorouting', 'smart');
      | 
      | %Rearrange system
      | Simulink.BlockDiagram.arrangeSystem(gcb);
      | 
      | %Refresh
      | treeValues = FailureInjectionPointHelper.getAllFmAndParamsAsTreeString(gcb);
      | mo = Simulink.Mask.get(gcb);
      | dc = mo.getDialogControl('GbFmInfo');
      | treeView = dc.getDialogControl('TreeViewFM');
      | treeView.TreeItems = {};
      | treeView.TreeItems = treeValues;
      mask DialogControl TreeViewFM Prompt: Failure Mode Information
      mask DialogControl BtnOpen Prompt: Open FIP
      mask DialogControl BtnOpen Callback: open_system(gcb,'force');
      mask DialogControl BtnNew Prompt: New
      mask DialogControl BtnNew Callback:
      | dialog_fipManager_single(gcb, '');
      | 
      | %Enable move, edit, delete buttons
      | mo = Simulink.Mask.get(gcb);
      | mo.getDialogControl('BtnMoveUp').Enabled = 'on';
      | mo.getDialogControl('BtnMoveDown').Enabled = 'on';
      | mo.getDialogControl('BtnEdit').Enabled = 'on';
      | mo.getDialogControl('BtnDelete').Enabled = 'on';
      mask DialogControl BtnEdit Prompt: Edit
      mask DialogControl BtnEdit Callback:
      | mo = Simulink.Mask.get(gcb);
      | dc = mo.getDialogControl('GbFmInfo');
      | treeView = dc.getDialogControl('TreeViewFM');
      | try
      |     a = treeView.getSelectedItems();
      |     p = split(a, '/');
      | catch
      |     return;
      | end
      | dialog_fipManager_single(gcb, p{1});
      mask DialogControl BtnDelete Prompt: Delete
      mask DialogControl BtnDelete Callback:
      | %Get name of the failure mode block
      | mo = Simulink.Mask.get(gcb);
      | dc = mo.getDialogControl('GbFmInfo');
      | treeView = dc.getDialogControl('TreeViewFM');
      | try
      |     a = treeView.getSelectedItems();
      |     p = split(a, '/'); %name of failure mode block is p{1}
      | catch
      |     return;
      | end
      | 
      | %Save outport handle of the last and inport handle of the next block
      | lh = get_param([gcb,'/',p{1}],'LineHandles');
      | last_out = get_param(lh.Inport(1),'SrcPortHandle');
      | next_in = get_param(lh.Outport(1),'DstPortHandle');
      | 
      | %Delete connecting lines and failure mode block
      | delete_line(lh.Inport(1));
      | delete_line(lh.Outport(1));
      | fm_handle = get_param([gcb,'/',p{1}],'Handle');
      | delete_block(fm_handle);
      | 
      | % Generate new line from outport last to inport next
      | add_line(gcb, last_out, next_in, 'autorouting', 'smart');
      | 
      | %Rearrange system
      | Simulink.BlockDiagram.arrangeSystem(gcb);
      | 
      | %Disable move, edit, delete buttons in case all FMs are deleted
      | last_block = get_param(last_out,'Parent');
      | last_is_inport = strcmp(get_param(last_block,'BlockType'),'Inport');
      | next_block = get_param(next_in,'Parent');
      | next_is_outport = strcmp(get_param(next_block,'BlockType'),'Outport');
      | if (last_is_inport && next_is_outport)
      |     mo.getDialogControl('BtnMoveUp').Enabled = 'off';
      |     mo.getDialogControl('BtnMoveDown').Enabled = 'off';
      |     mo.getDialogControl('BtnEdit').Enabled = 'off';
      |     mo.getDialogControl('BtnDelete').Enabled = 'off';
      | end
      | 
      | %Refresh
      | treeValues = FailureInjectionPointHelper.getAllFmAndParamsAsTreeString(gcb);
      | mo = Simulink.Mask.get(gcb);
      | dc = mo.getDialogControl('GbFmInfo');
      | treeView = dc.getDialogControl('TreeViewFM');
      | treeView.TreeItems = {};
      | treeView.TreeItems = treeValues;
      mask DialogControl BtnRefresh Prompt: Refresh
      mask DialogControl BtnRefresh Callback:
      | set_param(gcb,'LinkStatus','none');
      | 
      | treeValues = FailureInjectionPointHelper.getAllFmAndParamsAsTreeString(gcb);
      | mo = Simulink.Mask.get(gcb);
      | dc = mo.getDialogControl('GbFmInfo');
      | treeView = dc.getDialogControl('TreeViewFM');
      | treeView.TreeItems = {};
      | treeView.TreeItems = treeValues;
      mask Display: image('icons/failure_injection_point.png','center')
  Detect Change : simulink/Logic and Bit Operations/Detect Change  vinit=0  OutDataTypeStr=boolean
  Trigger FIP : LibFaultInjectionControls/Trigger FIP  Active=off  MaintenanceTask=1  RiskTime=1  FailureRate=1.0E-3  isDSF=off  DSFjson=JSON
      settings: SourceProductName=Fault Injection Controls
  analog Switch : Stateflow chart  TreatAsAtomicUnit=on
  Out1 : Outport
  wires:
  Detect Change/1 -> analog Switch/1(handleStateChanged)
  In1/1 -> Detect Change/1
  analog Switch/1(analogSwitchState) -> Out1/1
  Trigger FIP/1 -> analog Switch/2(fail)
